simulink model "CubaModelLQR"  (R2016a)
settings: Solver=FixedStepAuto  SolverMode=SingleTasking  StartTime=0.0  StopTime=5  FixedStep=0.001  RelTol=1e-3
values from neighbouring files (symbols this model uses):
  C_K = 2.1e-3    (= 0.0021)    [LQR_Calculation.m]
  C_R = 2.1268e-5    (= 2.1268e-05)    [LQR_Calculation.m]
  g = 9.81    [LQR_Calculation.m]
  l_AB = 0.08455    [LQR_Calculation.m]
  l_SA = 0.0751442    [LQR_Calculation.m]
  m_K = 0.294    [LQR_Calculation.m]
  m_R = 0.1298    [LQR_Calculation.m]
  O_G_A = O_K_A + m_R * l_AB^2    (= 0.0042279015845)    [LQR_Calculation.m]
  O_R_B = 0.088e-3    (= 8.8e-05)    [LQR_Calculation.m]
  phi_K0 = degtorad(0)    [LQR_Calculation.m]
  phi_K__d0 = degtorad(0)    [LQR_Calculation.m]
  phi_R0 = degtorad(0)    [LQR_Calculation.m]
  phi_R__d0 = degtorad(0)    [LQR_Calculation.m]
  T_M_m = 12.4e-3    (= 0.0124)    [LQR_Calculation.m]
undefined symbols (not defined in the file or in its folder): K
settings Model: Creator=michael  LastModifiedBy=ich

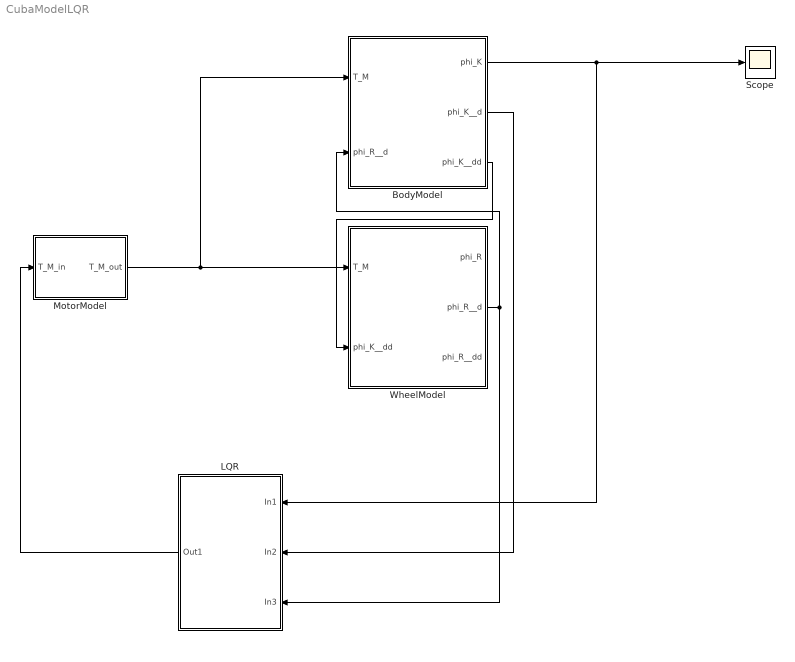
== system CubaModelLQR ==
  BodyModel : Subsystem  SystemSampleTime=0.001
  LQR : Subsystem  SystemSampleTime=0.02
  "MotorModel " : Subsystem
  Scope : Scope
  WheelModel : Subsystem  SystemSampleTime=0.001
  wires:
  BodyModel/3(phi_K__dd) -> WheelModel/2(phi_K__dd)
  "MotorModel "/1(T_M_out) -> BodyModel/1(T_M), WheelModel/1(T_M)
  BodyModel/1(phi_K) -> LQR/1(In1), Scope/1
  BodyModel/2(phi_K__d) -> LQR/2(In2)
  WheelModel/2(phi_R__d) -> LQR/3(In3), BodyModel/2(phi_R__d)
  LQR/1(Out1) -> "MotorModel "/1(T_M_in)

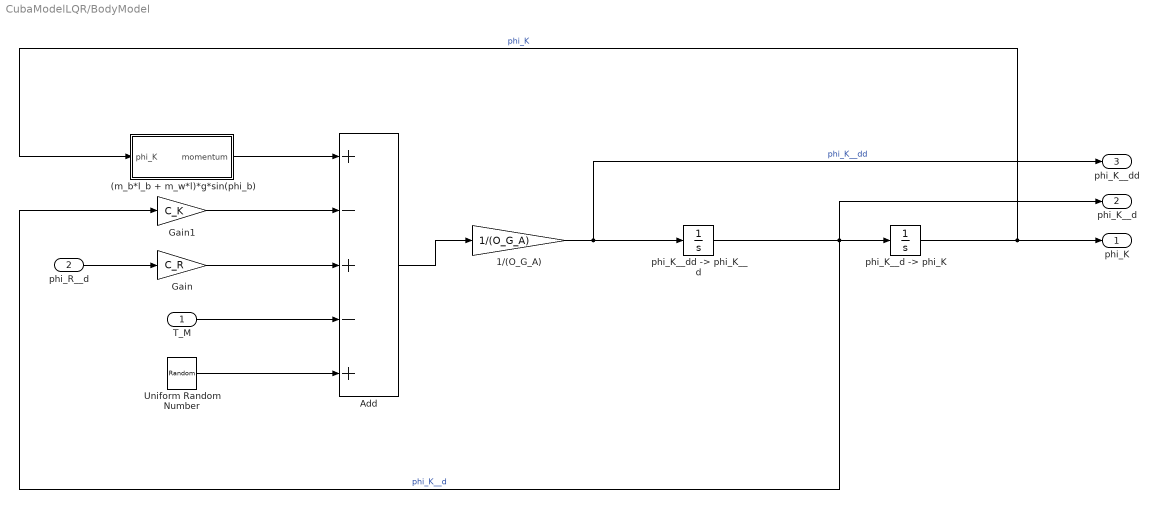
== system CubaModelLQR/BodyModel ==
  T_M : Inport
  phi_R__d : Inport  Port=2
  (m_b*l_b + m_w*l)*g*sin(phi_b) : Subsystem
  1/(O_G_A) : Gain  Gain=1/(O_G_A)
  Add : Sum  Inputs=+-+-+
  Gain : Gain  Gain=C_R
  Gain1 : Gain  Gain=C_K
  Uniform Random Number : UniformRandomNumber  Minimum=-0.001  Maximum=0.001  SampleTime=0.001
  "phi_K__d -> phi_K" : Integrator  InitialCondition=phi_K0
  "phi_K__dd -> phi_K__d" : Integrator  InitialCondition=phi_K__d0
  phi_K : Outport
  phi_K__d : Outport  Port=2
  phi_K__dd : Outport  Port=3
  wires:
  T_M/1 -> Add/4
  Gain/1 -> Add/3
  Gain1/1 -> Add/2
  (m_b*l_b + m_w*l)*g*sin(phi_b)/1(momentum) -> Add/1
  phi_R__d/1 -> Gain/1
  Add/1 -> 1/(O_G_A)/1
  1/(O_G_A)/1 -> phi_K__dd/1, "phi_K__dd -> phi_K__d"/1  "phi_K__dd"
  "phi_K__dd -> phi_K__d"/1 -> Gain1/1, phi_K__d/1, "phi_K__d -> phi_K"/1  "phi_K__d"
  "phi_K__d -> phi_K"/1 -> phi_K/1, (m_b*l_b + m_w*l)*g*sin(phi_b)/1(phi_K)  "phi_K"
  Uniform Random Number/1 -> Add/5

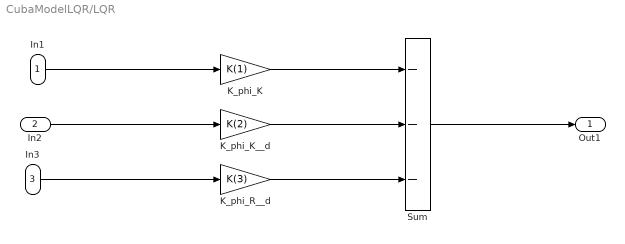
== system CubaModelLQR/LQR ==
  In1 : Inport
  In2 : Inport  Port=2
  In3 : Inport  Port=3
  K_phi_K : Gain  Gain=K(1)
  K_phi_K__d : Gain  Gain=K(2)
  K_phi_R__d : Gain  Gain=K(3)
  Sum : Sum  Inputs=---
  Out1 : Outport
  wires:
  In1/1 -> K_phi_K/1
  In3/1 -> K_phi_R__d/1
  In2/1 -> K_phi_K__d/1
  Sum/1 -> Out1/1
  K_phi_K/1 -> Sum/1
  K_phi_K__d/1 -> Sum/2
  K_phi_R__d/1 -> Sum/3

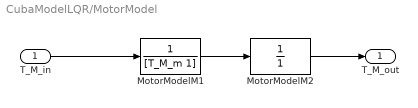
== system CubaModelLQR/MotorModel  ==
  T_M_in : Inport
  MotorModelM1 : TransferFcn  Denominator=[T_M_m 1]
  MotorModelM2 : TransferFcn  Denominator=[0 1]
  T_M_out : Outport
  wires:
  T_M_in/1 -> MotorModelM1/1
  MotorModelM1/1 -> MotorModelM2/1
  MotorModelM2/1 -> T_M_out/1

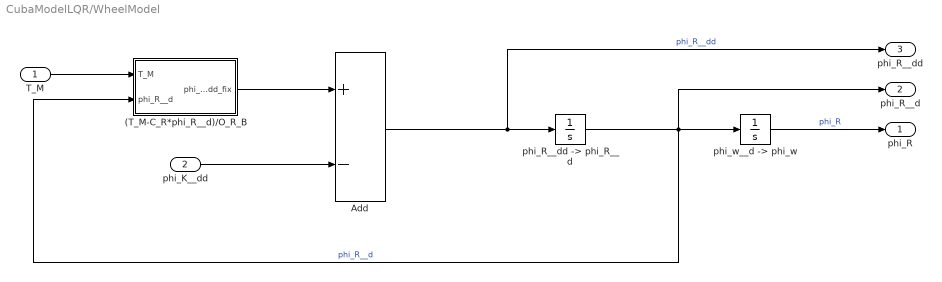
== system CubaModelLQR/WheelModel ==
  T_M : Inport
  phi_K__dd : Inport  Port=2
  (T_M-C_R*phi_R__d)/O_R_B : Subsystem
  Add : Sum  Inputs=+-
  "phi_R__dd -> phi_R__d" : Integrator  InitialCondition=phi_R__d0
  "phi_w__d -> phi_w" : Integrator  InitialCondition=phi_R0
  phi_R : Outport
  phi_R__d : Outport  Port=2
  phi_R__dd : Outport  Port=3
  wires:
  phi_K__dd/1 -> Add/2
  Add/1 -> phi_R__dd/1, "phi_R__dd -> phi_R__d"/1  "phi_R__dd"
  "phi_R__dd -> phi_R__d"/1 -> phi_R__d/1, (T_M-C_R*phi_R__d)/O_R_B/2(phi_R__d), "phi_w__d -> phi_w"/1  "phi_R__d"
  (T_M-C_R*phi_R__d)/O_R_B/1(phi_R__dd_fix) -> Add/1
  T_M/1 -> (T_M-C_R*phi_R__d)/O_R_B/1(T_M)
  "phi_w__d -> phi_w"/1 -> phi_R/1  "phi_R"

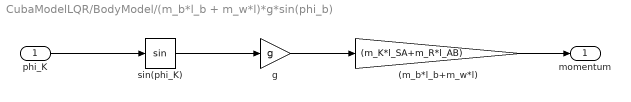
== system CubaModelLQR/BodyModel/(m_b*l_b + m_w*l)*g*sin(phi_b) ==
  phi_K : Inport
  (m_b*l_b+m_w*l) : Gain  Gain=(m_K*l_SA+m_R*l_AB)
  g : Gain  Gain=g
  sin(phi_K) : Trigonometry
  momentum : Outport
  wires:
  sin(phi_K)/1 -> g/1
  phi_K/1 -> sin(phi_K)/1
  g/1 -> (m_b*l_b+m_w*l)/1
  (m_b*l_b+m_w*l)/1 -> momentum/1

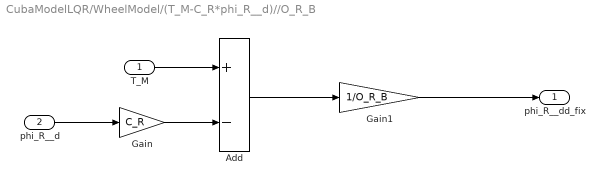
== system CubaModelLQR/WheelModel/(T_M-C_R*phi_R__d)//O_R_B ==
  T_M : Inport
  phi_R__d : Inport  Port=2
  Add : Sum  Inputs=+-
  Gain : Gain  Gain=C_R
  Gain1 : Gain  Gain=1/O_R_B
  phi_R__dd_fix : Outport
  wires:
  T_M/1 -> Add/1
  phi_R__d/1 -> Gain/1
  Gain/1 -> Add/2
  Add/1 -> Gain1/1
  Gain1/1 -> phi_R__dd_fix/1
